simulink model "Mennaaa"  (R2016a)
settings: Solver=VariableStepAuto  StartTime=0.0  StopTime=10.0  RelTol=1e-3
values from neighbouring files (symbols this model uses):
  A = [ 0 1 0 0 0 0 0 0 ; -(k1+k2)/m1 -(c1+c2)/m1 0 0 k2/m1 c2/m1 -k2*l1/m1 -c2*l1/m1 ; 0 0 0 1 0 0 0 0 ; 0 0 -(k1+k2)/m2 -(c1+c2)/m2 k2/m2 c2/m2 k2*l2/m2 c2*l2/m2 ; 0 0 0 0 0 1 0 0 ; k2/m c2/m k2/m c2/m 2*k2/m 2*c2/m (k2*l1-k2*l2)/m (c1*l2-c2*l2)/m ; 0 0 0 0 0 0 0 1; -k2*l1/J -c2*l1/J k2*l2/J c2*l2/J (k2*l1-k2*l2)/J (c2*l1-c2*l2)/J -(k2*l1^2+k2*l2^2)/J -(c2*l1^2+c2*l2^2)/J]    [Project01.m]
  B = [ 0 0 0 0 ; 1/m1 0 0 0 ; 0 0 0 0 ; 0 0 1/m2 0 ; 0 0 0 0 ; 0 0 0 0 ; 0 0 0 0 ; 0 0 0 0]    [Project01.m]
  C = [ 1 0 0 0 0 0 0 0 ; 0 0 1 0 0 0 0 0 ; 0 0 0 0 0 1 0 0 ; 0 0 0 0 0 0 0 1]    [Project01.m]
  D = [ 0 0 0 0 ; 0 0 0 0 ; 0 0 0 0 ; 0 0 0 0]    [Project01.m]
settings Model: Creator=star  LastModifiedBy=star

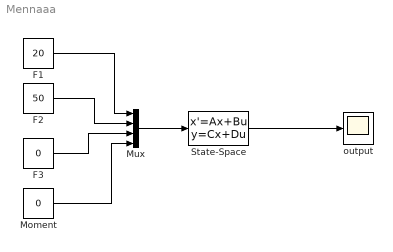
== system Mennaaa ==
  F1 : Constant  Value=20
  F2 : Constant  Value=50
  F3 : Constant  Value=0
  "Moment " : Constant  Value=0
  Mux : Mux
  State-Space : StateSpace  A=A  B=B  C=C  D=D  X0=[0 0 0 0 0 0 0 0]
  output : Scope
  wires:
  F2/1 -> Mux/2
  Mux/1 -> State-Space/1
  State-Space/1 -> output/1
  F1/1 -> Mux/1
  F3/1 -> Mux/3
  "Moment "/1 -> Mux/4
